simulink model "SiMoDronesMK"  (R2022a)
settings: Solver=FixedStepAuto  StartTime=0.0  StopTime=60  FixedStep=0.005  MaxStep=1e-3  MinStep=5e-5  RelTol=1e-5  AbsTol=1e-5  EnableMultiTasking=on
StopFcn:
  | save log.mat
  | [px4,optitrack,control,simulink]=traite_data_full('log.mat');
  | plot_data;
values from neighbouring files (symbols this model uses):
  aero =     [log.mat]
  drone =     [log.mat]
  dT_px4_udp = 0.02    [SimulationStartupScript.m]    (also in log.mat)
  dT_udp = 0.02    [SimulationStartupScript.m]    (also in log.mat)
  dT_udp_px4 = 0.02    [SimulationStartupScript.m]    (also in log.mat)
  Iload_UAVaxis = [0.00408625  0  0; 0  0.00408625  0; 0  0  8.625e-05]    [log.mat]
  init_state =     [log.mat]
  kpx = 1    [log.mat]
  kvx = 0.35    [log.mat]
  mass = 0.207    [log.mat]
  measure =     [log.mat]
  motor =     [log.mat]
  noisetrigger = 0    [log.mat]
  regul =     [log.mat]
  tdrop = 30    [SimulationStartupScript.m]    (also in log.mat)
  Te = 2e-2    (= 0.02)    [SimulationStartupScript.m]    (also in log.mat)
  th0 = 0.45    [log.mat]
  Ts_px4 = 5e-3    (= 0.005)    [SimulationStartupScript.m]    (also in log.mat)
undefined symbols (not defined in the file or in its folder): DiscIntNeverNeededParam, frame_t, gcbh, sigbuilder_block, sldrt_modeswitch, Standard_Devices, UDP_Protocol
libraries: simulink x11, orocomplib x9, vrlib x5, sldrtlib x4, sharedtransform x3, shared6dofsys x2, sharedutil x1, shared6dof x1, lib_isae_drones x1, simulink_need_slupdate x1, aerolibanimutils x1
(part 2 of 3)

== system SiMoDronesMK/Measurement block /Measure /optitrack ==
  pos_vel_NED : Inport
  att_eul_NED : Inport  Port=2
  Attitude optitrack : Subsystem
  XYZ optitrack : Subsystem
  pos_vel_optitrack : Outport
  att_eul_optitrack : Outport  Port=2
  wires:
  XYZ optitrack/1(pos_vel_optitrack) -> pos_vel_optitrack/1
  pos_vel_NED/1 -> XYZ optitrack/1(pos_vel_NED)
  att_eul_NED/1 -> Attitude optitrack/1(att_eul_NED)
  Attitude optitrack/1(att_eul_optitrack) -> att_eul_optitrack/1

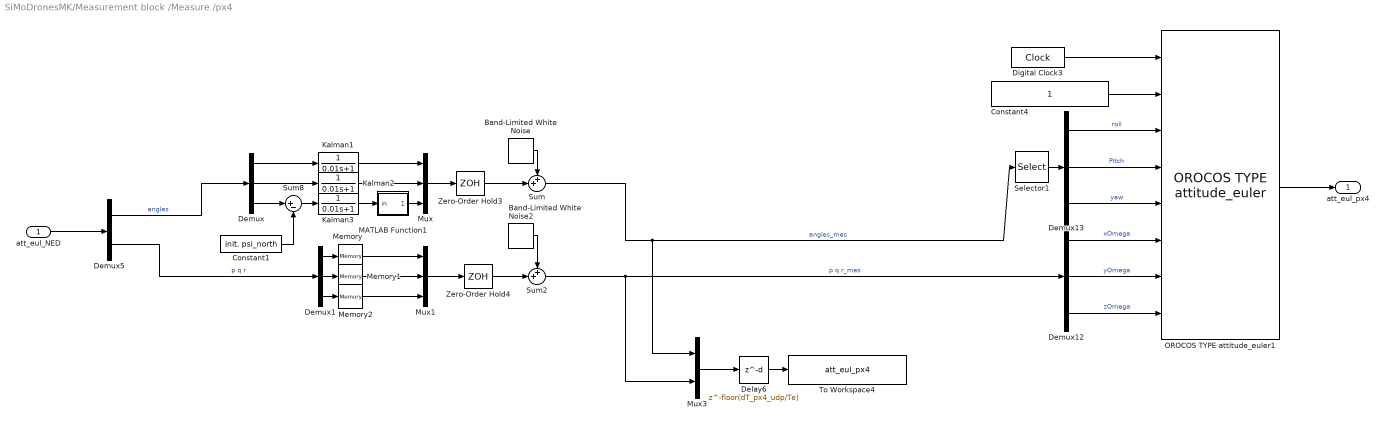
== system SiMoDronesMK/Measurement block /Measure /px4 ==
  att_eul_NED : Inport
  Band-Limited White Noise : simulink/Sources/Band-Limited White Noise  Cov=[measure.noise_power_angles]  Ts=Ts_px4  seed=[23341]
  Band-Limited White Noise2 : simulink/Sources/Band-Limited White Noise  Cov=[measure.noise_power_pqr]  Ts=Ts_px4  seed=[23341]
  Constant1 : Constant  Value=init. psi_north
  Constant4 : Constant  OutDataTypeStr=uint8  SampleTime=Ts_px4
  Delay6 : Delay  DelayLength=floor(dT_px4_udp/Te)  InitialCondition=0  SampleTime=Te
  Demux{,1,12..13} (4 alike) : Demux  Outputs=3
  Demux5 : Demux  Outputs=2
  Digital Clock3 : DigitalClock  SampleTime=Ts_px4
  Kalman1 : TransferFcn  Denominator=[0.01 1]
  Kalman2 : TransferFcn  Denominator=[0.01 1]
  Kalman3 : TransferFcn  Denominator=[0.01 1]
  MATLAB Function1 : MATLAB Function  TreatAsAtomicUnit=on
  Memory : Memory
  Memory1 : Memory
  Memory2 : Memory
  Mux : Mux  Inputs=3
  Mux1 : Mux  Inputs=3
  Mux3 : Mux  Inputs=2
  OROCOS TYPE attitude_euler1 : orocomplib/OROCOS TYPE attitude_euler
      settings: SourceProductName=Orocos Component Target
  Selector1 : Selector  InputPortWidth=3  IndexOptions=Index vector (dialog)  Indices=[1 2 3]  OutputSizes=1
  Sum : Sum  Inputs=++|
  Sum2 : Sum  Inputs=++|
  Sum8 : Sum  Inputs=|+-
  To Workspace4 : ToWorkspace  VariableName=att_eul_px4  SampleTime=Te
  Zero-Order Hold3 : ZeroOrderHold  SampleTime=Ts_px4
  Zero-Order Hold4 : ZeroOrderHold  SampleTime=Ts_px4
  att_eul_px4 : Outport
  wires:
  Delay6/1 -> To Workspace4/1
  Mux3/1 -> Delay6/1
  Demux13/2 -> OROCOS TYPE attitude_euler1/4  "Pitch"
  Constant4/1 -> OROCOS TYPE attitude_euler1/2
  Demux13/1 -> OROCOS TYPE attitude_euler1/3  "roll"
  Selector1/1 -> Demux13/1
  Demux13/3 -> OROCOS TYPE attitude_euler1/5  "yaw"
  Demux12/3 -> OROCOS TYPE attitude_euler1/8  "zOmega"
  Digital Clock3/1 -> OROCOS TYPE attitude_euler1/1
  Demux12/2 -> OROCOS TYPE attitude_euler1/7  "yOmega"
  Demux12/1 -> OROCOS TYPE attitude_euler1/6  "xOmega"
  OROCOS TYPE attitude_euler1/1 -> att_eul_px4/1
  Demux/3 -> Sum8/1
  Sum8/1 -> Kalman3/1
  Constant1/1 -> Sum8/2
  MATLAB Function1/1(out) -> Mux/3
  Memory2/1 -> Mux1/3
  Zero-Order Hold4/1 -> Sum2/2
  Zero-Order Hold3/1 -> Sum/2
  Mux1/1 -> Zero-Order Hold4/1
  Memory1/1 -> Mux1/2
  Memory/1 -> Mux1/1
  Demux1/3 -> Memory2/1
  Demux1/2 -> Memory1/1
  Demux1/1 -> Memory/1
  Kalman3/1 -> MATLAB Function1/1(in)
  Kalman2/1 -> Mux/2
  Kalman1/1 -> Mux/1
  Demux/2 -> Kalman2/1
  Demux/1 -> Kalman1/1
  Mux/1 -> Zero-Order Hold3/1
  Band-Limited White Noise2/1 -> Sum2/1
  Sum2/1 -> Demux12/1, Mux3/2  "p q r_mes"
  Demux5/2 -> Demux1/1  "p q r"
  Band-Limited White Noise/1 -> Sum/1
  Sum/1 -> Selector1/1, Mux3/1  "angles_mes"
  Demux5/1 -> Demux/1  "angles"
  att_eul_NED/1 -> Demux5/1

== system SiMoDronesMK/Measurement block /UDP link + Measure/Mesure ==
  pos_vel_opti : Inport
  att_eul_opti : Inport  Port=2
  att_eul_px4 : Inport  Port=3
  Bus Mapping1 : Subsystem
  Demux1 : Demux  Outputs=2
  Demux2 : Demux  Outputs=2
  Demux5 : Demux  Outputs=2
  pos_vel_optitrack : Outport
  att_eul_optitrack : Outport  Port=2
  att_eul_px4_ : Outport  Port=3
  wires:
  Demux2/1 -> Bus Mapping1/1(Position)  "Position_mes"
  Demux5/1 -> Bus Mapping1/3(Attitude)  "angles_mes"
  Demux5/2 -> Bus Mapping1/4(Omega)  "p q r"
  Demux2/2 -> Bus Mapping1/2(Velocity)  "vitesse_Re"
  Bus Mapping1/1(pos_vel_optitrack) -> pos_vel_optitrack/1
  Bus Mapping1/2(att_eul_optitrack) -> att_eul_optitrack/1
  pos_vel_opti/1 -> Demux2/1
  att_eul_opti/1 -> Demux5/1
  att_eul_px4/1 -> Demux1/1
  Demux1/1 -> Bus Mapping1/5(Att_px4)
  Bus Mapping1/3(att_px4) -> att_eul_px4_/1
  Demux1/2 -> Bus Mapping1/6(Omega_px4)  "p q r"

== system SiMoDronesMK/Measurement block /UDP link + Measure/UDP link ==
  Subsystem4 : Subsystem
  pos_vel_optitrack : Outport
  att_eul_optitrack : Outport  Port=2
  att_eul_px4 : Outport  Port=3
  wires:
  Subsystem4/1(pos_vel_optitrack) -> pos_vel_optitrack/1
  Subsystem4/2(att_eul_px4) -> att_eul_px4/1
  Subsystem4/3(att_eul_optitrack) -> att_eul_optitrack/1

== system SiMoDronesMK/Position Control1/X control/Controller1 ==
  Xr : Inport
  X : Inport  Port=2
  Vx : Inport  Port=3
  Adaptive  PI : Subsystem
  Adaptive PI : Subsystem
  Add : Sum  Inputs=+-
  Add2 : Sum  Inputs=+-
  Gain : Gain  Gain=-1
  Gain1 : Gain  Gain=-1
  Gain2 : Gain  Gain=-1
  Saturation1 : Saturate  UpperLimit=2  LowerLimit=-2
  Theta_tgt : Outport
  wires:
  X/1 -> Gain1/1
  Vx/1 -> Gain2/1
  Adaptive  PI/1(PD Out) -> Theta_tgt/1
  Add/1 -> Adaptive PI/1(X error)
  Adaptive PI/1(PI Out) -> Add2/1
  Add2/1 -> Saturation1/1
  Saturation1/1 -> Adaptive  PI/1(Vx Error)
  Gain/1 -> Add/1
  Gain1/1 -> Add/2
  Gain2/1 -> Add2/2
  Xr/1 -> Gain/1

== system SiMoDronesMK/Position Control1/Y  control/Controller ==
  Yr : Inport
  Y : Inport  Port=2
  Vy : Inport  Port=3
  Adaptive  PI : Subsystem
  Adaptive PI : Subsystem
  Add : Sum  Inputs=+-
  Add2 : Sum  Inputs=+-
  Saturation1 : Saturate  UpperLimit=2  LowerLimit=-2
  Roll_tgt : Outport
  wires:
  Y/1 -> Add/2
  Vy/1 -> Add2/2
  Adaptive  PI/1(PD Out) -> Roll_tgt/1
  Add/1 -> Adaptive PI/1(Y error)
  Adaptive PI/1(PI Out) -> Add2/1
  Add2/1 -> Saturation1/1
  Saturation1/1 -> Adaptive  PI/1(Vy Error)
  Yr/1 -> Add/1

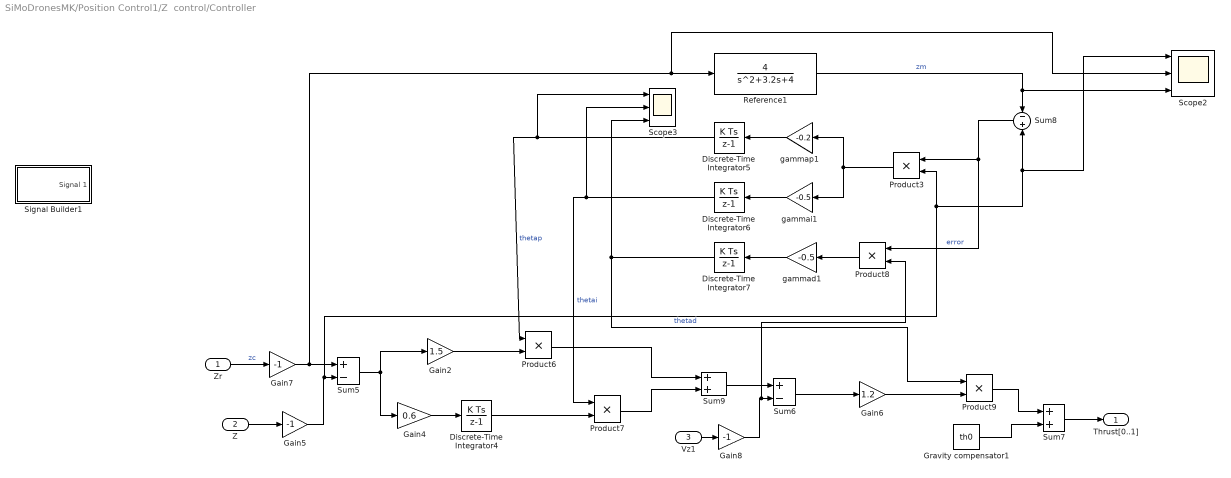
== system SiMoDronesMK/Position Control1/Z  control/Controller ==
  Zr : Inport
  Z : Inport  Port=2
  Vz1 : Inport  Port=3
  Discrete-Time Integrator{4..7} (4 alike) : DiscreteIntegrator  InitialCondition=1  SampleTime=0.02  ICPrevOutput=DiscIntNeverNeededParam  ICPrevScaledInput=DiscIntNeverNeededParam
  Gain2 : Gain  Gain=1.5
  Gain4 : Gain  Gain=0.6
  Gain5 : Gain  Gain=-1
  Gain6 : Gain  Gain=1.2
  Gain7 : Gain  Gain=-1
  Gain8 : Gain  Gain=-1
  Gravity compensator1 : Constant  Value=th0
  Product{3,6..9} (5 alike) : Product
  Reference1 : TransferFcn  Numerator=[4]  Denominator=[1 3.2 4]
  Scope2 : Scope  NumInputPorts=3
  Scope3 : Scope  NumInputPorts=3
  Signal Builder1 : Subsystem  Tag=STV Subsys  LoadFcn=sigbuilder_block('load');  StartFcn=sigbuilder_block('start');  StopFcn=sigbuilder_block('stop');  ClipboardFcn=sigbuilder_block('clipboard');  mask(Sigbuilder block){tuvar=[0:10]}
      mask help: Simulink:masks:SigbuilderBlock_MD
      mask init:
      | if ~strcmp(get_param(bdroot(gcbh),'SimulationStatus'),'stopped') tuvar = sigbuilder_block('maskInit'); end
      settings: CopyFcn=sigbuilder_block('copy');  DeleteFcn=sigbuilder_block('delete');  ModelCloseFcn=sigbuilder_block('modelClose');  PreSaveFcn=sigbuilder_block('preSave');  PauseFcn=sigbuilder_block('pause');  ContinueFcn=sigbuilder_block('continue');  NameChangeFcn=sigbuilder_block('namechange');  OpenFcn=sigbuilder_block('open',[437.6 199.2 550.4 400 ]);  CloseFcn=sigbuilder_block('close');
      mask Display: plot(0, 0, 100, 100,[2, 2, 32, 32, 2], [68, 8, 8, 68, 68],[32, 2], [38, 38], [32, 19, 2],[53, 60, 44], [32, 17, 17, 2],[16, 16, 31, 31]);txt = getActiveGroup(gcbh);text(2, 100, txt,'verticalAlignment', 'top');
  Sum5 : Sum  Inputs=+-
  Sum6 : Sum  Inputs=+-
  Sum7 : Sum
  Sum8 : Sum  Inputs=-+
  Sum9 : Sum
  gammad1 : Gain  Gain=-0.5
  gammai1 : Gain  Gain=-0.5
  gammap1 : Gain  Gain=-0.2
  Thrust[0..1] : Outport
  wires:
  Gain5/1 -> Scope2/1, Sum8/2, Product3/2, Sum5/2
  Discrete-Time Integrator7/1 -> Scope3/3, Product9/1  "thetad"
  Product3/1 -> gammai1/1, gammap1/1
  Zr/1 -> Gain7/1  "zc"
  Discrete-Time Integrator5/1 -> Scope3/1, Product6/1  "thetap"
  Gain8/1 -> Product8/2, Sum6/2
  Product7/1 -> Sum9/2
  gammap1/1 -> Discrete-Time Integrator5/1
  Sum6/1 -> Gain6/1
  Gain2/1 -> Product6/2
  Gain6/1 -> Product9/2
  gammai1/1 -> Discrete-Time Integrator6/1
  Discrete-Time Integrator4/1 -> Product7/2
  gammad1/1 -> Discrete-Time Integrator7/1
  Product6/1 -> Sum9/1
  Vz1/1 -> Gain8/1
  Gravity compensator1/1 -> Sum7/2
  Sum9/1 -> Sum6/1
  Sum7/1 -> Thrust[0..1]/1
  Sum5/1 -> Gain4/1, Gain2/1
  Gain7/1 -> Scope2/2, Reference1/1, Sum5/1
  Z/1 -> Gain5/1
  Product8/1 -> gammad1/1
  Discrete-Time Integrator6/1 -> Scope3/2, Product7/1  "thetai"
  Product9/1 -> Sum7/1
  Gain4/1 -> Discrete-Time Integrator4/1
  Reference1/1 -> Sum8/1, Scope2/3  "zm"
  Sum8/1 -> Product8/1, Product3/1  "error"

== system SiMoDronesMK/Visu 3D/Simulink 3D/Coordinate Transformations ==
  att_eul : Inport
  pos_vel : Inport  Port=2
  Demux1 : Demux  Outputs=2
  Demux2 : Demux  Outputs=2
  Demux3 : Demux  Outputs=3
  Demux4 : Demux  Outputs=3
  Gain : Gain  Gain=[1 1 -1 1]
  Gain1 : Gain  Gain=[1 1 -1]
  Gain3 : Gain  Gain=-1
  Math Function : Math  Operator=transpose  SignedPower=on
  Mux : Mux  Inputs=3
  Mux2 : Mux  Inputs=3
  Rotation Angles to Direction Cosine Matrix1 : sharedtransform/Rotation Angles to Direction Cosine Matrix  rotationOrder=XYZ  aMode=aMode
      settings: SourceProductBaseCode=AE,PW,DR,MT,VE
  Rotation Matrix to VRML Rotation : vrlib/Utilities/Rotation Matrix to VR Rotation  maxzero=1e-5
      settings: SourceProductBaseCode=SL
  Terminator : Terminator
  Terminator1 : Terminator
  VR Signal Expander : vrlib/VR Signal Expander  outwidth=4  outidx=[1 3 2 4]
  VR Signal Expander1 : vrlib/VR Signal Expander  outwidth=3  outidx=[1 3 2]
  VR Signal Expander2 : vrlib/VR Signal Expander  outwidth=4  outidx=[4]
  CameraFollowRotation : Outport
  CameraFollowTranslation : Outport  Port=2
  orientation : Outport  Port=3
  position : Outport  Port=4
  wires:
  att_eul/1 -> Demux1/1
  Demux1/2 -> Terminator1/1
  Demux1/1 -> Demux4/1  "Position"
  pos_vel/1 -> Demux2/1
  Demux2/2 -> Terminator/1
  Demux2/1 -> Demux3/1  "Position"
  Demux3/2 -> Mux2/2
  Demux3/1 -> Mux2/1
  Demux4/2 -> Mux/2
  Demux4/3 -> Mux/3
  Demux4/1 -> Mux/1
  Gain3/1 -> VR Signal Expander2/1
  VR Signal Expander2/1 -> CameraFollowRotation/1
  Demux3/3 -> Mux2/3, Gain3/1
  VR Signal Expander1/1 -> CameraFollowTranslation/1, position/1  "pos_VRML"
  Gain/1 -> VR Signal Expander/1
  Rotation Matrix to VRML Rotation/1 -> Gain/1
  Math Function/1 -> Rotation Matrix to VRML Rotation/1  "DCM_Body_2_NED"
  Rotation Angles to Direction Cosine Matrix1/1 -> Math Function/1  "DCM_NED_2_Body"
  Mux/1 -> Rotation Angles to Direction Cosine Matrix1/1
  Gain1/1 -> VR Signal Expander1/1  "pos_ENU"
  Mux2/1 -> Gain1/1  "pos_NED"
  VR Signal Expander/1 -> orientation/1

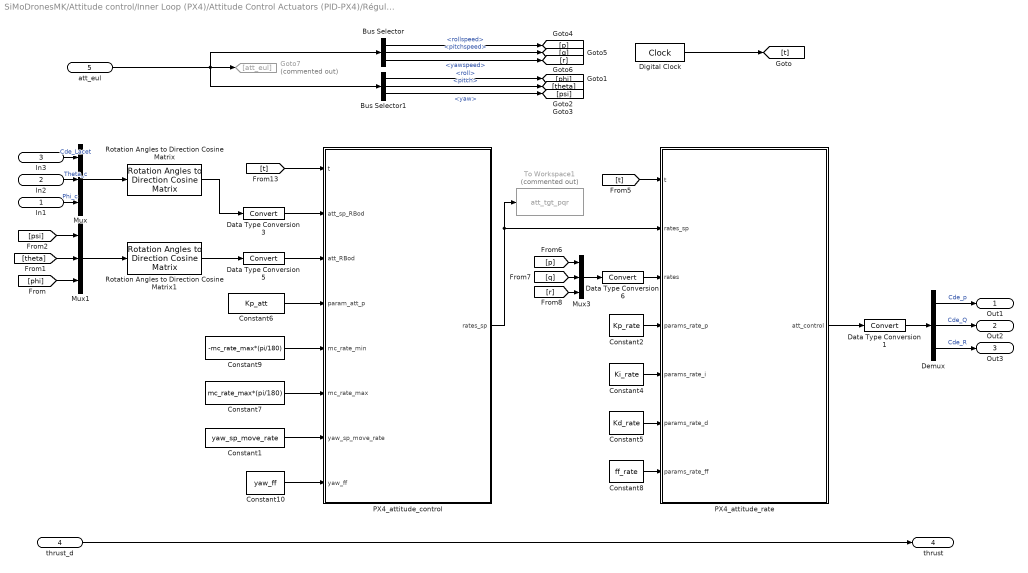
== system SiMoDronesMK/Attitude control/Inner Loop (PX4)/Attitude Control Actuators (PID-PX4)/Régulations ==
  In1 : Inport
  In2 : Inport  Port=2
  In3 : Inport  Port=3
  thrust_d : Inport  Port=4
  att_eul : Inport  Port=5
  Bus Selector : BusSelector  OutputSignals=rollspeed,pitchspeed,yawspeed
  Bus Selector1 : BusSelector  OutputSignals=roll,pitch,yaw
  Constant1 : Constant  Value=yaw_sp_move_rate  OutDataTypeStr=Inherit: Inherit via back propagation  SampleTime=-1
  Constant10 : Constant  Value=yaw_ff  OutDataTypeStr=Inherit: Inherit via back propagation  SampleTime=-1
  Constant2 : Constant  Value=Kp_rate  OutDataTypeStr=Inherit: Inherit via back propagation  SampleTime=-1
  Constant4 : Constant  Value=Ki_rate  OutDataTypeStr=Inherit: Inherit via back propagation  SampleTime=-1
  Constant5 : Constant  Value=Kd_rate  OutDataTypeStr=Inherit: Inherit via back propagation  SampleTime=-1
  Constant6 : Constant  Value=Kp_att  OutDataTypeStr=Inherit: Inherit via back propagation  SampleTime=-1
  Constant7 : Constant  Value=mc_rate_max*(pi/180)  OutDataTypeStr=Inherit: Inherit via back propagation  SampleTime=-1
  Constant8 : Constant  Value=ff_rate  OutDataTypeStr=Inherit: Inherit via back propagation  SampleTime=-1
  Constant9 : Constant  Value=-mc_rate_max*(pi/180)  OutDataTypeStr=Inherit: Inherit via back propagation  SampleTime=-1
  Data Type Conversion{1,3,5..6} (4 alike) : DataTypeConversion  SaturateOnIntegerOverflow=off  LockScale=on
  Demux : Demux  Outputs=3
  Digital Clock : DigitalClock  SampleTime=-1
  Goto7 : Goto  Commented=on  GotoTag=att_eul
  Mux : Mux  Inputs=3
  Mux1 : Mux  Inputs=3
  Mux3 : Mux  Inputs=3
  PX4_attitude_control : MATLAB Function  TreatAsAtomicUnit=on
  PX4_attitude_rate : MATLAB Function  TreatAsAtomicUnit=on
  Rotation Angles to Direction Cosine Matrix : sharedtransform/Rotation Angles to Direction Cosine Matrix  rotationOrder=ZYX  aMode=aMode
      settings: SourceProductBaseCode=AE,PW,DR,MT,VE
  Rotation Angles to Direction Cosine Matrix1 : sharedtransform/Rotation Angles to Direction Cosine Matrix  rotationOrder=ZYX  aMode=aMode
      settings: SourceProductBaseCode=AE,PW,DR,MT,VE
  To Workspace1 : ToWorkspace  Commented=on  VariableName=att_tgt_pqr  SampleTime=Te
  Out1 : Outport
  Out2 : Outport  Port=2
  Out3 : Outport  Port=3
  thrust : Outport  Port=4
  wires:
  Data Type Conversion1/1 -> Demux/1
  Demux/3 -> Out3/1  "Cde_R"
  Demux/2 -> Out2/1  "Cde_Q"
  Demux/1 -> Out1/1  "Cde_p"
  PX4_attitude_rate/1(att_control) -> Data Type Conversion1/1
  [phi] -> Mux1/3
  [psi] -> Mux1/1
  Mux1/1 -> Rotation Angles to Direction Cosine Matrix1/1
  In1/1 -> Mux/3  "Phi_c"
  In2/1 -> Mux/2  "Theta_c"
  In3/1 -> Mux/1  "Cde_Lacet"
  Mux/1 -> Rotation Angles to Direction Cosine Matrix/1
  Constant10/1 -> PX4_attitude_control/8(yaw_ff)
  Constant7/1 -> PX4_attitude_control/6(mc_rate_max)
  Constant9/1 -> PX4_attitude_control/5(mc_rate_min)
  Constant6/1 -> PX4_attitude_control/4(param_att_p)
  Bus Selector1/3 -> [psi]  "<yaw>"
  Bus Selector1/1 -> [phi]  "<roll>"
  Bus Selector1/2 -> [theta]  "<pitch>"
  Bus Selector/1 -> [p]  "<rollspeed>"
  Bus Selector/2 -> [q]  "<pitchspeed>"
  Bus Selector/3 -> [r]  "<yawspeed>"
  thrust_d/1 -> thrust/1
  Digital Clock/1 -> [t]
  att_eul/1 -> Bus Selector1/1, Bus Selector/1, Goto7/1
  Data Type Conversion3/1 -> PX4_attitude_control/2(att_sp_RBod)
  Data Type Conversion5/1 -> PX4_attitude_control/3(att_RBod)
  PX4_attitude_control/1(rates_sp) -> PX4_attitude_rate/2(rates_sp), To Workspace1/1
  Constant1/1 -> PX4_attitude_control/7(yaw_sp_move_rate)
  [r] -> Mux3/3
  [q] -> Mux3/2
  [p] -> Mux3/1
  Mux3/1 -> Data Type Conversion6/1
  [t] -> PX4_attitude_rate/1(t)
  Constant2/1 -> PX4_attitude_rate/4(params_rate_p)
  Constant4/1 -> PX4_attitude_rate/5(params_rate_i)
  Constant5/1 -> PX4_attitude_rate/6(params_rate_d)
  Constant8/1 -> PX4_attitude_rate/7(params_rate_ff)
  Data Type Conversion6/1 -> PX4_attitude_rate/3(rates)
  [theta] -> Mux1/2
  [t] -> PX4_attitude_control/1(t)
  Rotation Angles to Direction Cosine Matrix1/1 -> Data Type Conversion5/1
  Rotation Angles to Direction Cosine Matrix/1 -> Data Type Conversion3/1

== system SiMoDronesMK/Attitude control/Udp send/send_udp/QUADRI_EDU1 ==
  note: QUADRI EDU 1
  float : Inport
  Int : Inport  Port=2
  Packet Output2 : sldrtlib/Packet Output  SampleTime=Te  MaxMissedTicks=10  ShowMissedTicks=off  YieldWhenWaiting=off  DrvName=Standard_Devices/UDP_Protocol  DrvAddress=9000  DrvOptions=[184509651 9000]  PacketSize=8+50*4+50*2  DataTypes={'2*int32','50*single','50*int16'}  ShowReady=off  ShowError=off  PacketID=1  ByteOrder=1  InitialValue=[]  FinalValue=[]
      settings: AttributesFormatString=Standard Devices\nUDP Protocol [2328h]
  wires:
  Int/1 -> Packet Output2/3
  float/1 -> Packet Output2/2

== system SiMoDronesMK/Attitude control/Udp send/send_udp/QUADRI_EDU2 ==
  note: QUADRI EDU 2
  float : Inport
  Int : Inport  Port=2
  Packet Output3 : sldrtlib/Packet Output  SampleTime=Te  MaxMissedTicks=10  ShowMissedTicks=off  YieldWhenWaiting=off  DrvName=Standard_Devices/UDP_Protocol  DrvAddress=9000  DrvOptions=[184509652 9000]  PacketSize=8+50*4+50*2  DataTypes={'2*int32','50*single','50*int16'}  ShowReady=off  ShowError=off  PacketID=1  ByteOrder=1  InitialValue=[]  FinalValue=[]
      settings: AttributesFormatString=Standard Devices\nUDP Protocol [2328h]
  wires:
  Int/1 -> Packet Output3/3
  float/1 -> Packet Output3/2

== system SiMoDronesMK/Attitude control/Udp send/send_udp/QUADRI_EDU3 ==
  note: QUADRI EDU 3
  float : Inport
  Int : Inport  Port=2
  Packet Output1 : sldrtlib/Packet Output  SampleTime=Te  MaxMissedTicks=10  ShowMissedTicks=off  YieldWhenWaiting=off  DrvName=Standard_Devices/UDP_Protocol  DrvAddress=9000  DrvOptions=[184509570 9000]  PacketSize=8+50*4+50*2  DataTypes={'2*int32','50*single','50*int16'}  ShowReady=off  ShowError=off  PacketID=1  ByteOrder=1  InitialValue=[]  FinalValue=[]
      settings: AttributesFormatString=Standard Devices\nUDP Protocol [2328h]
  wires:
  Int/1 -> Packet Output1/3
  float/1 -> Packet Output1/2

== system SiMoDronesMK/Mass Change Model/Model/Acutators/Motor1 ==
  PWM : Inport
  Vbat : Inport  Port=2
  Mikrokopter drive : Subsystem  AncestorBlock=lib_isae_drones_1/Mavion drive  mask{coef_t2w=motor.coef_t2w, coef_delta_t2w=motor.coef_delta_t2w, coef_w2I=motor.coef_w2I, coef_delta_w2I=motor.coef_delta_w2I, Tau=motor.tr_mot, pourcentage=motor.pourcentage, omega_0=motor.w0, omega_max=motor.wmax, V_nom=motor.nominal_voltage}
      mask prompts: coef_t2w "PWM polynomial coefficients"; coef_delta_t2w "Delta(PWM) polynomial coefficients"; coef_w2I "Polynomial coefficients of the Propeller's rotationnal speed and the current relation"; coef_delta_w2I "Delta (Current - Propeller's rotationnal speed) polynomial coefficients"; Tau "Close loop Time constant (s)"; pourcentage "Close loop Time constant Variation (%)"; omega_0 "Initial rotationnal speed (rad/s)"; omega_max "Maximal rotationnal Speed (rad/s)"; V_nom "Nominal Motor Voltage (Volt)"
  Propeller : Subsystem
  Scope of  the mass : Scope
  speed : Outport
  Thrust : Outport  Port=2
  Torque : Outport  Port=3
  current : Outport  Port=4
  wires:
  Mikrokopter drive/1(w(rad/s)) -> Propeller/1(w (rad/s)), speed/1
  Vbat/1 -> Mikrokopter drive/2(Vbat)
  Propeller/2(Torque (N.m)) -> Torque/1
  Mikrokopter drive/2(I (Amps)) -> current/1
  Propeller/1(Thrust (N)) -> Scope of  the mass/1, Thrust/1
  PWM/1 -> Mikrokopter drive/1(PWM (0..1))

== system SiMoDronesMK/Mass Change Model/Model/Acutators/Motor2 ==
  PWM : Inport
  Vbat : Inport  Port=2
  Mikrokopter drive : Subsystem  AncestorBlock=lib_isae_drones_1/Mavion drive  mask{coef_t2w=motor.coef_t2w, coef_delta_t2w=motor.coef_delta_t2w, coef_w2I=motor.coef_w2I, coef_delta_w2I=motor.coef_delta_w2I, Tau=motor.tr_mot, pourcentage=motor.pourcentage, omega_0=motor.w0, omega_max=motor.wmax, V_nom=motor.nominal_voltage}
      mask prompts: coef_t2w "PWM polynomial coefficients"; coef_delta_t2w "Delta(PWM) polynomial coefficients"; coef_w2I "Polynomial coefficients of the Propeller's rotationnal speed and the current relation"; coef_delta_w2I "Delta (Current - Propeller's rotationnal speed) polynomial coefficients"; Tau "Close loop Time constant (s)"; pourcentage "Close loop Time constant Variation (%)"; omega_0 "Initial rotationnal speed (rad/s)"; omega_max "Maximal rotationnal Speed (rad/s)"; V_nom "Nominal Motor Voltage (Volt)"
  Propeller : Subsystem
  speed : Outport
  Thrust : Outport  Port=2
  Torque : Outport  Port=3
  current : Outport  Port=4
  wires:
  PWM/1 -> Mikrokopter drive/1(PWM (0..1))
  Propeller/1(Thrust (N)) -> Thrust/1
  Mikrokopter drive/2(I (Amps)) -> current/1
  Propeller/2(Torque (N.m)) -> Torque/1
  Vbat/1 -> Mikrokopter drive/2(Vbat)
  Mikrokopter drive/1(w(rad/s)) -> speed/1, Propeller/1(w (rad/s))

== system SiMoDronesMK/Mass Change Model/Model/Acutators/Motor3 ==
  PWM : Inport
  Vbat : Inport  Port=2
  Mikrokopter drive : Subsystem  AncestorBlock=lib_isae_drones_1/Mavion drive  mask{coef_t2w=motor.coef_t2w, coef_delta_t2w=motor.coef_delta_t2w, coef_w2I=motor.coef_w2I, coef_delta_w2I=motor.coef_delta_w2I, Tau=motor.tr_mot, pourcentage=motor.pourcentage, omega_0=motor.w0, omega_max=motor.wmax, V_nom=motor.nominal_voltage}
      mask prompts: coef_t2w "PWM polynomial coefficients"; coef_delta_t2w "Delta(PWM) polynomial coefficients"; coef_w2I "Polynomial coefficients of the Propeller's rotationnal speed and the current relation"; coef_delta_w2I "Delta (Current - Propeller's rotationnal speed) polynomial coefficients"; Tau "Close loop Time constant (s)"; pourcentage "Close loop Time constant Variation (%)"; omega_0 "Initial rotationnal speed (rad/s)"; omega_max "Maximal rotationnal Speed (rad/s)"; V_nom "Nominal Motor Voltage (Volt)"
  Propeller : Subsystem
  speed : Outport
  Thrust : Outport  Port=2
  Torque : Outport  Port=3
  current : Outport  Port=4
  wires:
  Mikrokopter drive/1(w(rad/s)) -> Propeller/1(w (rad/s)), speed/1
  Vbat/1 -> Mikrokopter drive/2(Vbat)
  Propeller/2(Torque (N.m)) -> Torque/1
  Mikrokopter drive/2(I (Amps)) -> current/1
  Propeller/1(Thrust (N)) -> Thrust/1
  PWM/1 -> Mikrokopter drive/1(PWM (0..1))

== system SiMoDronesMK/Mass Change Model/Model/Acutators/Motor4 ==
  PWM : Inport
  Vbat : Inport  Port=2
  Mikrokopter drive : Subsystem  AncestorBlock=lib_isae_drones_1/Mavion drive  mask{coef_t2w=motor.coef_t2w, coef_delta_t2w=motor.coef_delta_t2w, coef_w2I=motor.coef_w2I, coef_delta_w2I=motor.coef_delta_w2I, Tau=motor.tr_mot, pourcentage=motor.pourcentage, omega_0=motor.w0, omega_max=motor.wmax, V_nom=motor.nominal_voltage}
      mask prompts: coef_t2w "PWM polynomial coefficients"; coef_delta_t2w "Delta(PWM) polynomial coefficients"; coef_w2I "Polynomial coefficients of the Propeller's rotationnal speed and the current relation"; coef_delta_w2I "Delta (Current - Propeller's rotationnal speed) polynomial coefficients"; Tau "Close loop Time constant (s)"; pourcentage "Close loop Time constant Variation (%)"; omega_0 "Initial rotationnal speed (rad/s)"; omega_max "Maximal rotationnal Speed (rad/s)"; V_nom "Nominal Motor Voltage (Volt)"
  Propeller : Subsystem
  speed : Outport
  Thrust : Outport  Port=2
  Torque : Outport  Port=3
  current : Outport  Port=4
  wires:
  PWM/1 -> Mikrokopter drive/1(PWM (0..1))
  Propeller/1(Thrust (N)) -> Thrust/1
  Mikrokopter drive/2(I (Amps)) -> current/1
  Propeller/2(Torque (N.m)) -> Torque/1
  Vbat/1 -> Mikrokopter drive/2(Vbat)
  Mikrokopter drive/1(w(rad/s)) -> speed/1, Propeller/1(w (rad/s))

== system SiMoDronesMK/Mass Change Model/Model/Acutators/Subsystem ==
  In1 : Inport
  In2 : Inport  Port=2
  In3 : Inport  Port=3
  In13 : Inport  Port=4
  In4 : Inport  Port=5
  In5 : Inport  Port=6
  In6 : Inport  Port=7
  In7 : Inport  Port=8
  In8 : Inport  Port=9
  In9 : Inport  Port=10
  In10 : Inport  Port=11
  In11 : Inport  Port=12
  In12 : Inport  Port=13
  In14 : Inport  Port=14
  In15 : Inport  Port=15
  In16 : Inport  Port=16
  Bus Creator{,1..4} (5 alike) : BusCreator  Inputs=4
  actuators : Outport
  wires:
  In12/1 -> Bus Creator4/1  "speed"
  In16/1 -> Bus Creator4/4  "current"
  In14/1 -> Bus Creator4/2  "thrust"
  In15/1 -> Bus Creator4/3  "torque"
  In8/1 -> Bus Creator3/1  "speed"
  In11/1 -> Bus Creator3/4  "current"
  In9/1 -> Bus Creator3/2  "thrust"
  In10/1 -> Bus Creator3/3  "torque"
  In4/1 -> Bus Creator2/1  "speed"
  In7/1 -> Bus Creator2/4  "current"
  In5/1 -> Bus Creator2/2  "thrust"
  In6/1 -> Bus Creator2/3  "torque"
  In1/1 -> Bus Creator1/1  "speed"
  In13/1 -> Bus Creator1/4  "current"
  In2/1 -> Bus Creator1/2  "thrust"
  In3/1 -> Bus Creator1/3  "torque"
  Bus Creator4/1 -> Bus Creator/4  "motor4"
  Bus Creator1/1 -> Bus Creator/1  "motor1"
  Bus Creator2/1 -> Bus Creator/2  "motor2"
  Bus Creator3/1 -> Bus Creator/3  "motor3"
  Bus Creator/1 -> actuators/1

== system SiMoDronesMK/Mass Change Model/Model/Custom Variable Mass 6DOF (Euler Angles)/Determine Force, Mass & Inertia ==
  note: Inertia Change
  note: Mass Change
  Vb : Inport
  forces : Inport  Port=2
  "mass " : Inport  Port=3
  mdot : Inport  Port=4
  I : Inport  Port=5
  I_dot : Inport  Port=6
  Add{,1..3} (4 alike) : Sum
  Ground : Ground
  Idrop : Step  Time=tdrop  Before=[0 0 0;0 0 0;0 0 0]  After=-Iload_UAVaxis  SampleTime=0
  Inertia  Drop : Subsystem
  Mass  Drop : Subsystem
  Massdrop : Step  Time=tdrop  After=-mass  SampleTime=0
  Matrix Concatenation : Concatenate  Mode=Multidimensional array
  Product : Product  SaturateOnIntegerOverflow=on  OutDataTypeStr=Inherit: Same as first input
  Sum : Sum  Inputs=|+-  SaturateOnIntegerOverflow=on
  "forces " : Outport
  mass : Outport  Port=2
  "I, I_dot " : Outport  Port=3
  Out9 : Outport  Port=4
  wires:
  Ground/1 -> Out9/1
  Matrix Concatenation/1 -> "I, I_dot "/1
  I_dot/1 -> Add3/2
  forces/1 -> Sum/1
  Vb/1 -> Product/1
  Sum/1 -> "forces "/1
  Product/1 -> Sum/2
  "mass "/1 -> Add/2
  Add/1 -> mass/1
  mdot/1 -> Add1/1
  Add1/1 -> Product/2
  I/1 -> Add2/2
  Add2/1 -> Matrix Concatenation/1
  Massdrop/1 -> Add/1
  Mass  Drop/1(Out1) -> Add1/2
  Idrop/1 -> Add2/1
  Add3/1 -> Matrix Concatenation/2
  Inertia  Drop/1(Out2) -> Add3/1

== system SiMoDronesMK/Mass Change Model/Model/Custom Variable Mass 6DOF (Euler Angles)/Velocity Conversion ==
  in : Inport  Unit=m/s
  Unit Conversion : UnitConversion
  out : Outport  VectorParamsAs1DForOutWhenUnconnected=off
  wires:
  in/1 -> Unit Conversion/1
  Unit Conversion/1 -> out/1

== system SiMoDronesMK/Mass Change Model/Model/Custom Variable Mass 6DOF (Euler Angles)/Velocity Conversion1 ==
  in : Inport  Unit=m/s
  Unit Conversion : UnitConversion
  out : Outport  VectorParamsAs1DForOutWhenUnconnected=off
  wires:
  in/1 -> Unit Conversion/1
  Unit Conversion/1 -> out/1

== system SiMoDronesMK/Mass Change Model/Model/Custom Variable Mass 6DOF (Euler Angles)/transform to Inertial axes  ==
  x y z : Inport
  transform coefficients : Inport  Port=2
  Product : Product  Multiplication=Matrix(*)  InputSameDT=on  SaturateOnIntegerOverflow=on  OutDataTypeStr=Inherit: Same as first input
  Reshape1 : Reshape  OutputDimensionality=Column vector (2-D)
  Reshape2 : Reshape
  Ve : Outport  VectorParamsAs1DForOutWhenUnconnected=off
  wires:
  Product/1 -> Reshape2/1
  transform coefficients/1 -> Product/1
  x y z/1 -> Reshape1/1
  Reshape1/1 -> Product/2
  Reshape2/1 -> Ve/1

== system SiMoDronesMK/Mass Change Model/Model/Quad rotor model1/Modèle Forces ==
  In1 : Inport
  In2 : Inport  Port=2
  In3 : Inport  Port=3
  In4 : Inport  Port=4
  vel1 : Inport  Port=5
  drone_mass_variable : Inport  Port=6
  Calcul Trainée Linéaire : Subsystem
  Coefficient de Poussée : Gain  Gain=Pw
  Math Function{,1..3} (4 alike) : Math  Operator=square  SignedPower=on
  Matrix Multiply : Product  Multiplication=Matrix(*)
  Mux : Mux  Inputs=2
  Orientation de la Poussée : Gain  Gain=-1
  Poids : Constant  Value=[0 0 g]  OutDataTypeStr=Inherit: Inherit via back propagation
  Poids1 : Constant  Value=[0 0]  OutDataTypeStr=Inherit: Inherit via back propagation
  Product : Product
  Sum : Sum  Inputs=++++
  Sum2 : Sum  Inputs=+++
  Out1 : Outport
  wires:
  Math Function2/1 -> Sum/2
  Math Function1/1 -> Sum/4
  Math Function/1 -> Sum/1
  Math Function3/1 -> Sum/3
  Orientation de la Poussée/1 -> Mux/2
  Calcul Trainée Linéaire/1(Trainée) -> Sum2/3  "trainee_lin_Rb"
  vel1/1 -> Calcul Trainée Linéaire/1(Vitesse_Rd)  "vitesse_Rb"
  Matrix Multiply/1 -> Sum2/2  "Poids_Rb"
  [DCM] -> Matrix Multiply/1
  Sum2/1 -> Out1/1  "F_Rb"
  Mux/1 -> Sum2/1  "Poussee_Rb"
  Poids1/1 -> Mux/1
  Coefficient de Poussée/1 -> Orientation de la Poussée/1
  Sum/1 -> Coefficient de Poussée/1
  In1/1 -> Math Function/1  "w1"
  In2/1 -> Math Function2/1  "w2"
  In3/1 -> Math Function3/1  "w3"
  In4/1 -> Math Function1/1  "w4"
  drone_mass_variable/1 -> Product/1
  Poids/1 -> Product/2  "Poids_Re"
  Product/1 -> Matrix Multiply/2

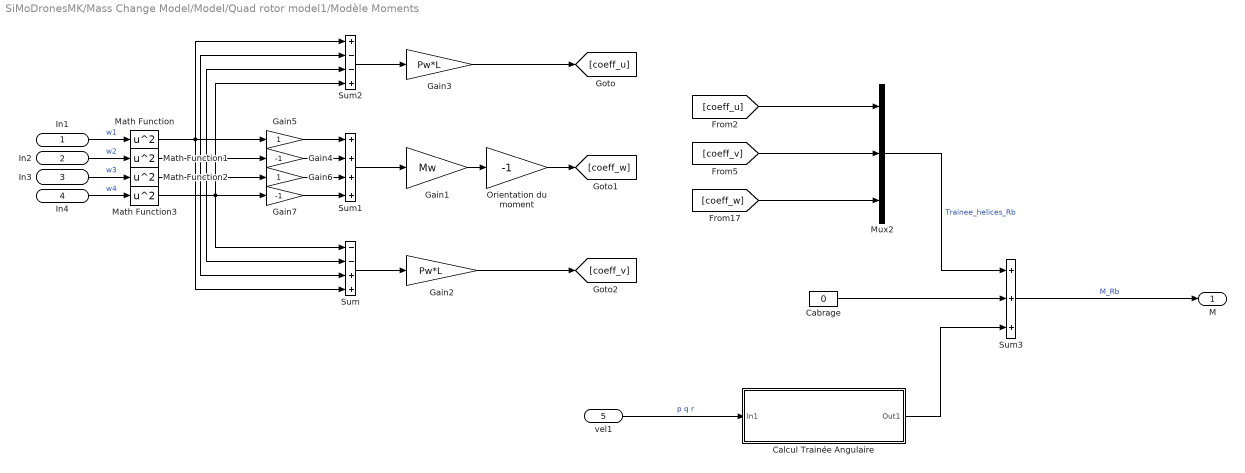
== system SiMoDronesMK/Mass Change Model/Model/Quad rotor model1/Modèle Moments ==
  In1 : Inport
  In2 : Inport  Port=2
  In3 : Inport  Port=3
  In4 : Inport  Port=4
  vel1 : Inport  Port=5
  Cabrage : Constant  Value=0
  Calcul Trainée Angulaire : Subsystem
  Gain1 : Gain  Gain=Mw
  Gain2 : Gain  Gain=Pw*L
  Gain3 : Gain  Gain=Pw*L
  Gain4 : Gain  Gain=-1
  Gain5 : Gain
  Gain6 : Gain
  Gain7 : Gain  Gain=-1
  Math Function{,1..3} (4 alike) : Math  Operator=square  SignedPower=on
  Mux2 : Mux  Inputs=3
  Orientation du moment : Gain  Gain=-1
  Sum : Sum  Inputs=--++
  Sum1 : Sum  Inputs=++++
  Sum2 : Sum  Inputs=+--+
  Sum3 : Sum  Inputs=+++
  M : Outport
  wires:
  Math Function3/1 -> Sum2/4, Sum/1, Gain7/1
  Math Function2/1 -> Sum2/3, Gain6/1, Sum/2
  Math Function1/1 -> Sum2/2, Sum/3, Gain4/1
  Math Function/1 -> Sum2/1, Sum/4, Gain5/1
  Orientation du moment/1 -> [coeff_w]
  Cabrage/1 -> Sum3/2
  Gain6/1 -> Sum1/3
  Gain5/1 -> Sum1/1
  [coeff_u] -> Mux2/1
  [coeff_v] -> Mux2/2
  Gain3/1 -> [coeff_u]
  Gain2/1 -> [coeff_v]
  Calcul Trainée Angulaire/1(Out1) -> Sum3/3
  vel1/1 -> Calcul Trainée Angulaire/1(In1)  "p q r"
  Mux2/1 -> Sum3/1  "Trainee_helices_Rb"
  Sum3/1 -> M/1  "M_Rb"
  [coeff_w] -> Mux2/3
  Gain7/1 -> Sum1/4
  Gain4/1 -> Sum1/2
  Gain1/1 -> Orientation du moment/1
  Sum1/1 -> Gain1/1
  Sum/1 -> Gain2/1
  Sum2/1 -> Gain3/1
  In3/1 -> Math Function2/1  "w3"
  In4/1 -> Math Function3/1  "w4"
  In2/1 -> Math Function1/1  "w2"
  In1/1 -> Math Function/1  "w1"

== system SiMoDronesMK/Measurement block /Measure /optitrack/Attitude optitrack ==
  att_eul_NED : Inport
  Band-Limited White Noise5 : simulink/Sources/Band-Limited White Noise  Cov=[measure.noise_power_angles]  Ts=Te  seed=[23341]
  Band-Limited White Noise6 : simulink/Sources/Band-Limited White Noise  Cov=[measure.noise_power_pqr]  Ts=Te  seed=[23341]
  Constant3 : Constant  OutDataTypeStr=uint8  SampleTime=Te
  Delay3 : Delay  DelayLength=floor(dT_udp/Te)  InitialCondition=init_state.Angles0  SampleTime=Te
  Delay4 : Delay  DelayLength=floor(dT_udp/Te)  InitialCondition=init_state.pqr0  SampleTime=Te
  Demux{6..7,10..11} (4 alike) : Demux  Outputs=3
  Demux2 : Demux  Outputs=2
  Digital Clock2 : DigitalClock  SampleTime=Te
  MATLAB Function : MATLAB Function  TreatAsAtomicUnit=on
  Mux1 : Mux  Inputs=2
  Mux2 : Mux  Inputs=3
  Mux5 : Mux  Inputs=3
  OROCOS TYPE attitude_euler : orocomplib/OROCOS TYPE attitude_euler
      settings: SourceProductName=Orocos Component Target
  Selector : Selector  InputPortWidth=3  IndexOptions=Index vector (dialog)  Indices=[1 2 3]  OutputSizes=1
  Sum6 : Sum  Inputs=++|
  Sum7 : Sum  Inputs=++|
  To Workspace1 : ToWorkspace  VariableName=att_eul_optitrack  SampleTime=Te
  att_eul_optitrack : Outport
  wires:
  Mux1/1 -> To Workspace1/1
  Demux2/2 -> Demux7/1
  Demux2/1 -> Demux6/1
  Demux11/3 -> OROCOS TYPE attitude_euler/5  "yaw"
  Demux11/2 -> OROCOS TYPE attitude_euler/4  "Pitch"
  Demux10/3 -> OROCOS TYPE attitude_euler/8  "zOmega"
  Demux11/1 -> OROCOS TYPE attitude_euler/3  "roll"
  Selector/1 -> Demux11/1
  Constant3/1 -> OROCOS TYPE attitude_euler/2
  Digital Clock2/1 -> OROCOS TYPE attitude_euler/1
  Demux10/1 -> OROCOS TYPE attitude_euler/6  "xOmega"
  Demux10/2 -> OROCOS TYPE attitude_euler/7  "yOmega"
  Mux5/1 -> Delay4/1
  Mux2/1 -> Delay3/1
  OROCOS TYPE attitude_euler/1 -> att_eul_optitrack/1
  MATLAB Function/1(out) -> Mux2/3
  Demux6/3 -> MATLAB Function/1(in)
  Sum7/1 -> Demux10/1, Mux1/2  "p q r_mes"
  Delay4/1 -> Sum7/2
  Delay3/1 -> Sum6/2
  Demux7/3 -> Mux5/3
  Demux7/2 -> Mux5/2
  Demux7/1 -> Mux5/1
  Demux6/2 -> Mux2/2
  Demux6/1 -> Mux2/1
  Band-Limited White Noise6/1 -> Sum7/1
  Band-Limited White Noise5/1 -> Sum6/1
  Sum6/1 -> Selector/1, Mux1/1  "angles_mes"
  att_eul_NED/1 -> Demux2/1

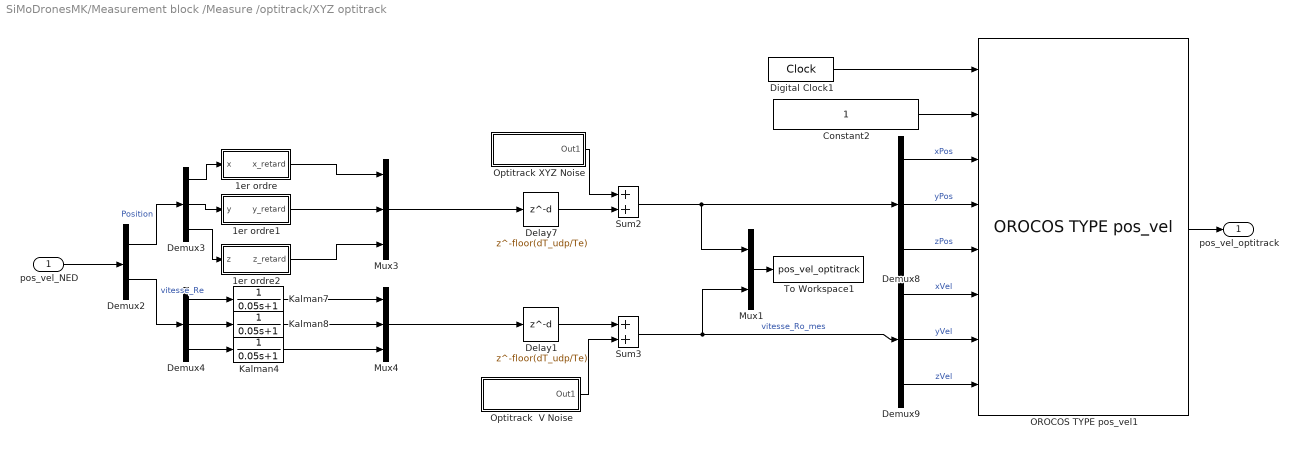
== system SiMoDronesMK/Measurement block /Measure /optitrack/XYZ optitrack ==
  pos_vel_NED : Inport
  1er ordre : Subsystem  mask{tr5=0.007, K=1, init_inte=init_state.Pterre0(1)}
      mask prompts: tr5 "Tau"; K "Gain Statique"; init_inte "Initialisation 1/p"
  1er ordre1 : Subsystem  mask{tr5=0.007, K=1, init_inte=init_state.Pterre0(2)}
      mask prompts: tr5 "Tau"; K "Gain Statique"; init_inte "Initialisation 1/p"
  1er ordre2 : Subsystem  mask{tr5=0.05, K=1, init_inte=init_state.Pterre0(3)}
      mask prompts: tr5 "Tau"; K "Gain Statique"; init_inte "Initialisation 1/p"
  Constant2 : Constant  OutDataTypeStr=uint8  SampleTime=Te
  Delay1 : Delay  DelayLength=floor(dT_udp/Te)  InitialCondition=init_state.Vuvw0  SampleTime=Te
  Delay7 : Delay  DelayLength=floor(dT_udp/Te)  InitialCondition=init_state.Pterre0  SampleTime=Te
  Demux2 : Demux  Outputs=2
  Demux{3..4,8..9} (4 alike) : Demux  Outputs=3
  Digital Clock1 : DigitalClock  SampleTime=Te
  Kalman4 : TransferFcn  Denominator=[0.05 1]
  Kalman7 : TransferFcn  Denominator=[0.05 1]
  Kalman8 : TransferFcn  Denominator=[0.05 1]
  Mux1 : Mux  Inputs=2
  Mux3 : Mux  Inputs=3
  Mux4 : Mux  Inputs=3
  OROCOS TYPE pos_vel1 : orocomplib/OROCOS TYPE pos_vel
      settings: SourceProductName=Orocos Component Target
  Optitrack  V Noise : Subsystem
  Optitrack XYZ Noise : Subsystem
  Sum2 : Sum
  Sum3 : Sum
  To Workspace1 : ToWorkspace  VariableName=pos_vel_optitrack  SampleTime=Te
  pos_vel_optitrack : Outport
  wires:
  Mux1/1 -> To Workspace1/1
  Demux8/3 -> OROCOS TYPE pos_vel1/5  "zPos"
  Demux8/1 -> OROCOS TYPE pos_vel1/3  "xPos"
  Demux8/2 -> OROCOS TYPE pos_vel1/4  "yPos"
  Demux9/2 -> OROCOS TYPE pos_vel1/7  "yVel"
  Demux9/1 -> OROCOS TYPE pos_vel1/6  "xVel"
  Demux9/3 -> OROCOS TYPE pos_vel1/8  "zVel"
  Digital Clock1/1 -> OROCOS TYPE pos_vel1/1
  OROCOS TYPE pos_vel1/1 -> pos_vel_optitrack/1
  Constant2/1 -> OROCOS TYPE pos_vel1/2
  Mux4/1 -> Delay1/1
  Mux3/1 -> Delay7/1
  1er ordre2/1(z_retard) -> Mux3/3
  pos_vel_NED/1 -> Demux2/1
  Delay7/1 -> Sum2/2
  Kalman4/1 -> Mux4/3
  Demux4/3 -> Kalman4/1
  Kalman8/1 -> Mux4/2
  Kalman7/1 -> Mux4/1
  Demux4/2 -> Kalman8/1
  Demux4/1 -> Kalman7/1
  Demux3/3 -> 1er ordre2/1(z)
  1er ordre1/1(y_retard) -> Mux3/2
  1er ordre/1(x_retard) -> Mux3/1
  Demux3/2 -> 1er ordre1/1(y)
  Demux3/1 -> 1er ordre/1(x)
  Sum3/1 -> Mux1/2, Demux9/1  "vitesse_Ro_mes"
  Demux2/2 -> Demux4/1  "vitesse_Re"
  Demux2/1 -> Demux3/1  "Position"
  Sum2/1 -> Mux1/1, Demux8/1
  Delay1/1 -> Sum3/1
  Optitrack  V Noise/1(Out1) -> Sum3/2
  Optitrack XYZ Noise/1(Out1) -> Sum2/1

== system SiMoDronesMK/Measurement block /UDP link + Measure/Mesure/Bus Mapping1 ==
  Position : Inport
  Velocity : Inport  Port=2
  Attitude : Inport  Port=3
  Omega : Inport  Port=4
  Att_px4 : Inport  Port=5
  Omega_px4 : Inport  Port=6
  Constant1 : Constant  Value=frame_t.BODY_NED  OutDataTypeStr=Enum: frame_t  SampleTime=Te
  Constant2 : Constant  Value=frame_t.LOCAL_NED  OutDataTypeStr=Enum: frame_t  SampleTime=Te
  Constant3 : Constant  Value=frame_t.BODY_NED  OutDataTypeStr=Enum: frame_t  SampleTime=Te
  Demux{,1..5} (6 alike) : Demux  Outputs=3
  Digital Clock1 : DigitalClock  SampleTime=Te
  Digital Clock2 : DigitalClock  SampleTime=Te
  Digital Clock3 : DigitalClock  SampleTime=Te
  OROCOS TYPE attitude_euler : orocomplib/OROCOS TYPE attitude_euler
      settings: SourceProductName=Orocos Component Target
  OROCOS TYPE attitude_euler1 : orocomplib/OROCOS TYPE attitude_euler
      settings: SourceProductName=Orocos Component Target
  OROCOS TYPE pos_vel : orocomplib/OROCOS TYPE pos_vel
      settings: SourceProductName=Orocos Component Target
  Selector : Selector  InputPortWidth=3  IndexOptions=Index vector (dialog)  Indices=[1 2 3]  OutputSizes=1
  Selector1 : Selector  InputPortWidth=3  IndexOptions=Index vector (dialog)  Indices=[1 2 3]  OutputSizes=1
  pos_vel_optitrack : Outport
  att_eul_optitrack : Outport  Port=2
  att_px4 : Outport  Port=3
  wires:
  Demux3/2 -> OROCOS TYPE attitude_euler/4  "Pitch"
  Demux3/3 -> OROCOS TYPE attitude_euler/5  "yaw"
  Demux3/1 -> OROCOS TYPE attitude_euler/3  "roll"
  Demux/1 -> OROCOS TYPE pos_vel/3  "xPos"
  Demux/2 -> OROCOS TYPE pos_vel/4  "yPos"
  Demux/3 -> OROCOS TYPE pos_vel/5  "zPos"
  Demux1/1 -> OROCOS TYPE pos_vel/6  "xVel"
  Demux1/2 -> OROCOS TYPE pos_vel/7  "yVel"
  Demux1/3 -> OROCOS TYPE pos_vel/8  "zVel"
  Demux2/1 -> OROCOS TYPE attitude_euler/6  "xOmega"
  Demux2/2 -> OROCOS TYPE attitude_euler/7  "yOmega"
  Demux2/3 -> OROCOS TYPE attitude_euler/8  "zOmega"
  Selector/1 -> Demux3/1
  Position/1 -> Demux/1
  Velocity/1 -> Demux1/1
  Attitude/1 -> Selector/1
  OROCOS TYPE pos_vel/1 -> pos_vel_optitrack/1
  OROCOS TYPE attitude_euler/1 -> att_eul_optitrack/1
  Constant2/1 -> OROCOS TYPE pos_vel/2
  Digital Clock1/1 -> OROCOS TYPE pos_vel/1
  Digital Clock2/1 -> OROCOS TYPE attitude_euler/1
  Constant1/1 -> OROCOS TYPE attitude_euler/2
  Demux5/2 -> OROCOS TYPE attitude_euler1/4  "Pitch"
  Demux5/3 -> OROCOS TYPE attitude_euler1/5  "yaw"
  Demux5/1 -> OROCOS TYPE attitude_euler1/3  "roll"
  Demux4/1 -> OROCOS TYPE attitude_euler1/6  "xOmega"
  Demux4/2 -> OROCOS TYPE attitude_euler1/7  "yOmega"
  Demux4/3 -> OROCOS TYPE attitude_euler1/8  "zOmega"
  Selector1/1 -> Demux5/1
  Omega/1 -> Demux2/1
  Att_px4/1 -> Selector1/1
  OROCOS TYPE attitude_euler1/1 -> att_px4/1
  Digital Clock3/1 -> OROCOS TYPE attitude_euler1/1
  Constant3/1 -> OROCOS TYPE attitude_euler1/2
  Omega_px4/1 -> Demux4/1

== system SiMoDronesMK/Measurement block /UDP link + Measure/UDP link/Subsystem4 ==
  " trame3" : Display  Commented=on
  Float : Subsystem
  MATLAB Function : MATLAB Function  TreatAsAtomicUnit=on
  Packet Input : sldrtlib/Packet Input  SampleTime=0.005  MaxMissedTicks=10  ShowMissedTicks=off  YieldWhenWaiting=off  DrvName=Standard_Devices/UDP_Protocol  DrvAddress=9010  DrvOptions=[184509470 9020]  PacketSize=8+50*4+50*2  DataTypes={'2*int32','50*single','50*int16'}  ShowReady=off  ShowError=off  PacketID=1  ByteOrder=1  ShowTimestamp=off
      settings: AttributesFormatString=Standard Devices\nUDP Protocol [2332h]
  Rate Transition : RateTransition  OutPortSampleTime=Te
  Rate Transition1 : RateTransition  OutPortSampleTime=Te
  Terminator : Terminator
  To Workspace10 : ToWorkspace  Commented=on  VariableName=ramp_feedback  SampleTime=Te
  pos_vel_optitrack : Outport
  att_eul_px4 : Outport  Port=2
  att_eul_optitrack : Outport  Port=3
  tag scope: Num_trame=global, offboard_mode=global, ramp_feed=global, servo=global
  wires:
  Packet Input/1 -> [Num_trame]
  Packet Input/2 -> Rate Transition/1  "float"
  Packet Input/3 -> Rate Transition1/1  "int"
  MATLAB Function/1(ramp_feedback) -> [ramp_feed], To Workspace10/1
  Float/1(att_eul_px4) -> att_eul_px4/1
  Float/2(pos_vel_optitrack) -> pos_vel_optitrack/1, " trame3"/1
  Float/3(att_eul_optitrack) -> att_eul_optitrack/1
  Rate Transition/1 -> Float/1(Float)
  Rate Transition1/1 -> MATLAB Function/1(u)
  MATLAB Function/2(offboard_button) -> [offboard_mode]
  MATLAB Function/4(servo) -> [servo]
  MATLAB Function/3(motor_speed) -> Terminator/1

== system SiMoDronesMK/Position Control1/X control/Controller1/Adaptive  PI ==
  Vx Error : Inport
  Add3 : Sum
  Discrete-Time Integrator : DiscreteIntegrator  gainval=kivx  ExternalReset=rising  SampleTime=-1  ICPrevOutput=DiscIntNeverNeededParam  ICPrevScaledInput=DiscIntNeverNeededParam
  Kp2 : Gain  Gain=kvx
  PD Out : Outport
  wires:
  Add3/1 -> PD Out/1
  Discrete-Time Integrator/1 -> Add3/2
  Vx Error/1 -> Discrete-Time Integrator/1, Kp2/1
  [offboard_mode] -> Discrete-Time Integrator/2
  Kp2/1 -> Add3/1

== system SiMoDronesMK/Position Control1/X control/Controller1/Adaptive PI ==
  X error : Inport
  Add1 : Sum
  Discrete-Time Integrator : DiscreteIntegrator  gainval=kix  ExternalReset=rising  SampleTime=-1  ICPrevOutput=DiscIntNeverNeededParam  ICPrevScaledInput=DiscIntNeverNeededParam
  Kp : Gain  Gain=kpx
  PI Out : Outport
  wires:
  X error/1 -> Discrete-Time Integrator/1, Kp/1
  Add1/1 -> PI Out/1
  Kp/1 -> Add1/1
  Discrete-Time Integrator/1 -> Add1/2
  [offboard_mode] -> Discrete-Time Integrator/2

== system SiMoDronesMK/Position Control1/Y  control/Controller/Adaptive  PI ==
  Vy Error : Inport
  Add3 : Sum
  Discrete-Time Integrator : DiscreteIntegrator  gainval=kivx  ExternalReset=rising  SampleTime=-1  ICPrevOutput=DiscIntNeverNeededParam  ICPrevScaledInput=DiscIntNeverNeededParam
  Kp2 : Gain  Gain=kvx
  PD Out : Outport
  wires:
  Add3/1 -> PD Out/1
  Discrete-Time Integrator/1 -> Add3/2
  Vy Error/1 -> Discrete-Time Integrator/1, Kp2/1
  [offboard_mode] -> Discrete-Time Integrator/2
  Kp2/1 -> Add3/1

== system SiMoDronesMK/Position Control1/Y  control/Controller/Adaptive PI ==
  Y error : Inport
  Add1 : Sum
  Discrete-Time Integrator : DiscreteIntegrator  gainval=kix  ExternalReset=rising  SampleTime=-1  ICPrevOutput=DiscIntNeverNeededParam  ICPrevScaledInput=DiscIntNeverNeededParam
  Kp : Gain  Gain=kpx
  PI Out : Outport
  wires:
  Y error/1 -> Discrete-Time Integrator/1, Kp/1
  Add1/1 -> PI Out/1
  Kp/1 -> Add1/1
  Discrete-Time Integrator/1 -> Add1/2
  [offboard_mode] -> Discrete-Time Integrator/2

== system SiMoDronesMK/Position Control1/Z  control/Controller/Signal Builder1 ==
  Demux : Demux  Tag=STV Demux  Outputs=1
      settings: DisplayOption=none
  FromWs : FromWorkspace  Tag=STV FromWs  VariableName=tuvar
      SigBuilderData=|
      | common.afterFinalStr = 'Extrapolate'
      | common.sampleTime = 0
      | dataSet.timeRange = [0 37]
      | dataSet.name = 'Group 1'
      | sbobj.Groups.Name = 'Group 1'
      | sbobj.Groups.Signals.Name = 'Signal 1'
      | sbobj.Groups.Signals.XData = [0 1 1 11 11 21 31 37]
      | sbobj.Groups.Signals.YData = [0 0 1.5 1.5 2 2 0 0]
      | sbobj.Groups.TimeRange = [0 37]
  Signal 1 : Outport  Tag=STV Outport
  wires:
  Demux/1 -> Signal 1/1
  FromWs/1 -> Demux/1

== system SiMoDronesMK/Mass Change Model/Model/Acutators/Motor1/Mikrokopter drive ==
  PWM (0..1) : Inport  OutDataTypeStr=double  PortDimensions=1  SampleTime=0
  Vbat : Inport  Port=2  OutDataTypeStr=double  PortDimensions=1  SampleTime=0
  close loop model : Subsystem
  w(rad/s) : Outport  OutDataTypeStr=double  PortDimensions=1  SampleTime=0
  I (Amps) : Outport  Port=2  OutDataTypeStr=double  PortDimensions=1  SampleTime=0
  wires:
  PWM (0..1)/1 -> close loop model/1(PWM)
  Vbat/1 -> close loop model/2("Vbat ")
  close loop model/1(w (rad/s)) -> w(rad/s)/1
  close loop model/2(I (amps)) -> I (Amps)/1

== system SiMoDronesMK/Mass Change Model/Model/Acutators/Motor1/Propeller ==
  w (rad/s) : Inport
  Polynomial : Polyval  Coefs=motor.coef_w2C
  Polynomial1 : Polyval  Coefs=motor.coef_w2P
  Thrust (N) : Outport
  Torque (N.m) : Outport  Port=2
  wires:
  Polynomial1/1 -> Thrust (N)/1
  Polynomial/1 -> Torque (N.m)/1
  w (rad/s)/1 -> Polynomial/1, Polynomial1/1

== system SiMoDronesMK/Mass Change Model/Model/Acutators/Motor2/Mikrokopter drive ==
  PWM (0..1) : Inport  OutDataTypeStr=double  PortDimensions=1  SampleTime=0
  Vbat : Inport  Port=2  OutDataTypeStr=double  PortDimensions=1  SampleTime=0
  close loop model : Subsystem
  w(rad/s) : Outport  OutDataTypeStr=double  PortDimensions=1  SampleTime=0
  I (Amps) : Outport  Port=2  OutDataTypeStr=double  PortDimensions=1  SampleTime=0
  wires:
  PWM (0..1)/1 -> close loop model/1(PWM)
  Vbat/1 -> close loop model/2("Vbat ")
  close loop model/1(w (rad/s)) -> w(rad/s)/1
  close loop model/2(I (amps)) -> I (Amps)/1

== system SiMoDronesMK/Mass Change Model/Model/Acutators/Motor2/Propeller ==
  w (rad/s) : Inport
  Polynomial : Polyval  Coefs=motor.coef_w2C
  Polynomial1 : Polyval  Coefs=motor.coef_w2P
  Thrust (N) : Outport
  Torque (N.m) : Outport  Port=2
  wires:
  w (rad/s)/1 -> Polynomial1/1, Polynomial/1
  Polynomial/1 -> Torque (N.m)/1
  Polynomial1/1 -> Thrust (N)/1

== system SiMoDronesMK/Mass Change Model/Model/Acutators/Motor3/Mikrokopter drive ==
  PWM (0..1) : Inport  OutDataTypeStr=double  PortDimensions=1  SampleTime=0
  Vbat : Inport  Port=2  OutDataTypeStr=double  PortDimensions=1  SampleTime=0
  close loop model : Subsystem
  w(rad/s) : Outport  OutDataTypeStr=double  PortDimensions=1  SampleTime=0
  I (Amps) : Outport  Port=2  OutDataTypeStr=double  PortDimensions=1  SampleTime=0
  wires:
  PWM (0..1)/1 -> close loop model/1(PWM)
  Vbat/1 -> close loop model/2("Vbat ")
  close loop model/1(w (rad/s)) -> w(rad/s)/1
  close loop model/2(I (amps)) -> I (Amps)/1

== system SiMoDronesMK/Mass Change Model/Model/Acutators/Motor3/Propeller ==
  w (rad/s) : Inport
  Polynomial : Polyval  Coefs=motor.coef_w2C
  Polynomial1 : Polyval  Coefs=motor.coef_w2P
  Thrust (N) : Outport
  Torque (N.m) : Outport  Port=2
  wires:
  Polynomial1/1 -> Thrust (N)/1
  Polynomial/1 -> Torque (N.m)/1
  w (rad/s)/1 -> Polynomial/1, Polynomial1/1

== system SiMoDronesMK/Mass Change Model/Model/Acutators/Motor4/Mikrokopter drive ==
  PWM (0..1) : Inport  OutDataTypeStr=double  PortDimensions=1  SampleTime=0
  Vbat : Inport  Port=2  OutDataTypeStr=double  PortDimensions=1  SampleTime=0
  close loop model : Subsystem
  w(rad/s) : Outport  OutDataTypeStr=double  PortDimensions=1  SampleTime=0
  I (Amps) : Outport  Port=2  OutDataTypeStr=double  PortDimensions=1  SampleTime=0
  wires:
  PWM (0..1)/1 -> close loop model/1(PWM)
  Vbat/1 -> close loop model/2("Vbat ")
  close loop model/1(w (rad/s)) -> w(rad/s)/1
  close loop model/2(I (amps)) -> I (Amps)/1

== system SiMoDronesMK/Mass Change Model/Model/Acutators/Motor4/Propeller ==
  w (rad/s) : Inport
  Polynomial : Polyval  Coefs=motor.coef_w2C
  Polynomial1 : Polyval  Coefs=motor.coef_w2P
  Thrust (N) : Outport
  Torque (N.m) : Outport  Port=2
  wires:
  w (rad/s)/1 -> Polynomial1/1, Polynomial/1
  Polynomial/1 -> Torque (N.m)/1
  Polynomial1/1 -> Thrust (N)/1

== system SiMoDronesMK/Mass Change Model/Model/Custom Variable Mass 6DOF (Euler Angles)/Determine Force, Mass & Inertia/Inertia  Drop ==
  Add3 : Sum
  Step1 : Step  Time=tdrop  Before=[0 0 0;0 0 0;0 0 0]  After=-Iload_UAVaxis/0.02  SampleTime=0
  Step2 : Step  Time=tdrop  Before=[0 0 0;0 0 0;0 0 0]  After=Iload_UAVaxis/0.02  SampleTime=0
  Out2 : Outport
  wires:
  Step1/1 -> Add3/1
  Step2/1 -> Add3/2
  Add3/1 -> Out2/1

== system SiMoDronesMK/Mass Change Model/Model/Custom Variable Mass 6DOF (Euler Angles)/Determine Force, Mass & Inertia/Mass  Drop ==
  Add3 : Sum
  Step1 : Step  Time=tdrop  After=-mass/0.02  SampleTime=0
  Step2 : Step  Time=tdrop+0.02  After=mass/0.02  SampleTime=0
  Out1 : Outport
  wires:
  Step1/1 -> Add3/1
  Step2/1 -> Add3/2
  Add3/1 -> Out1/1

== system SiMoDronesMK/Mass Change Model/Model/Quad rotor model1/Modèle Forces/Calcul Trainée Linéaire ==
  Vitesse_Rd : Inport
  Demux : Demux  Outputs=3
  Demux1 : Demux  Outputs=3
  Gain : Gain  Gain=-1
  Gain2 : Gain  Gain=.5
  Gain3 : Gain  Gain=-1
  Gain4 : Gain  Gain=-1
  Math Function : Math  Operator=square  SignedPower=on
  Mux2 : Mux  Inputs=3
  Product{1..2,4..5} (4 alike) : Product  RndMeth=Zero
  Product3 : Product  Inputs=3  RndMeth=Zero
  Sign1 : Signum
  Sign2 : Signum
  Sign3 : Signum
  Surface : Constant  Value=S_drag_uvw  SampleTime=0
  density : Constant  Value=rho  SampleTime=0
  dragCoeff : Constant  Value=C_drag  SampleTime=0
  vel1 : InportShadow
  Trainée : Outport
  wires:
  Gain2/1 -> Product4/2
  Math Function/1 -> Product4/1
  Product4/1 -> Product3/1
  Vitesse_Rd/1 -> Math Function/1
  dragCoeff/1 -> Product3/3  "Cd"
  Surface/1 -> Product3/2
  density/1 -> Gain2/1
  Mux2/1 -> Trainée/1
  Product5/1 -> Gain4/1
  Product2/1 -> Gain3/1
  Product1/1 -> Gain/1
  vel1/1 -> Demux1/1
  Demux1/1 -> Sign2/1
  Demux1/2 -> Sign1/1
  Demux1/3 -> Sign3/1
  Sign2/1 -> Product1/1
  Sign1/1 -> Product2/1
  Sign3/1 -> Product5/1
  Demux/1 -> Product1/2
  Demux/2 -> Product2/2
  Demux/3 -> Product5/2
  Gain/1 -> Mux2/1
  Gain3/1 -> Mux2/2
  Gain4/1 -> Mux2/3
  Product3/1 -> Demux/1
